simulink model "atmoDrag"  (R2018b)
settings: Solver=VariableStepAuto  StartTime=0.0  StopTime=10.0  RelTol=1e-3
libraries: aerolibatmos2 x1
settings Model: Creator=willik50  LastModifiedBy=willik50

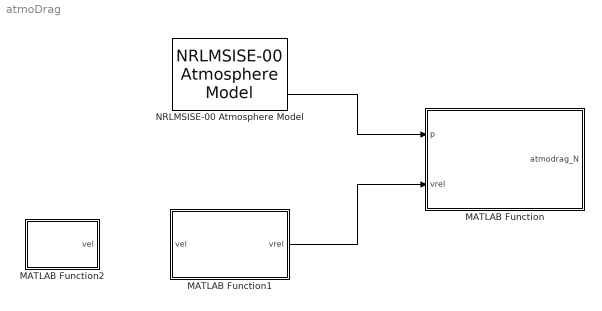
== system atmoDrag ==
  MATLAB Function : MATLAB Function  TreatAsAtomicUnit=on
  MATLAB Function1 : MATLAB Function  TreatAsAtomicUnit=on
  MATLAB Function2 : MATLAB Function  TreatAsAtomicUnit=on
  NRLMSISE-00 Atmosphere Model : aerolibatmos2/NRLMSISE-00 Atmosphere Model  units=Metric (MKS)  lst_input=off  flux_ap_input=off  flags_input=Internal  flags=ones(1,23)  oxygen_in=off  action=Warning
      settings: SourceProductName=Aerospace Blockset  SourceProductBaseCode=AE
  wires:
  NRLMSISE-00 Atmosphere Model/2 -> MATLAB Function/1(p)
  MATLAB Function1/1(vrel) -> MATLAB Function/2(vrel)

== matlab function atmoDrag/MATLAB Function1 ==
  data: vel input; vrel output
function vrel = relativeVelocity(vel)
%velocity relative to the atmosphere

%angula velocity of earth assumed to only be in z-direction despite wobble
%bc assumed to be very small, see pg 222 Rdot for x, y components
wx=0; %omega of earth in x direction
wy=0; %omega of earth in y direction

%vel in m/s, vrel in m/s
vrel = [diff(vel(1,1))+wy;diff(vel(2,1))-wx;diff(vel(3,1))];

== matlab function atmoDrag/MATLAB Function ==
  data: p input; atmodrag_N output; vrel input
function atmodrag_N = atmoDrag(p,vrel)
%Author Kate Williams
%Date created 2/21/2019
%function consists of basic atospheric equation

%drag in units of newtons, a 3D vector
%den=density, gathered from density model kg/m^3
%Cd = coeficent of drag, dimensionless
%A=exposed cross sectional area, m^2
%m=mass of cubsat, kg
%vrel= relative velocity m/s^2
%unitV= unit vector of relative velocity

%cubesat parameters
A= 0.1*0.1*2+0.1*0.3*4; %m^2 of a 3U cubesat
m=4; %kg, this is max mass allowed, final mass yet to be determined
Cd=2.2;% standard for 3U cubesat
%Cd = (1+2/3*sqrt(1-alpha)*sin(theta))*sin(theta)
%https://apps.dtic.mil/dtic/tr/fulltext/u2/a285118.pdf pg 16
%http://citeseerx.ist.psu.edu/viewdoc/download?doi=10.1.1.588.3019&rep=rep1&type=pdf

vrelMag=sqrt(sum(vrel.*vrel));
unitV=vrel/vrelMag; %direction of the drag

%below drag equation from vallado pg 551 eq8-28
atmodrag_N = -0.5*p*(Cd*A/m)*vrelMag^2*vrel*unitV; %drag occurs in opposite direction of velocity

== matlab function atmoDrag/MATLAB Function2 ==
  data: vel output
function vel = velocity()

vel = sqrt(GM?;
